simulink model "collision"  (R2018a)
settings: Solver=VariableStepAuto  StartTime=0.0  StopTime=120  FixedStep=0.01  MaxStep=.01  RelTol=1e-3
settings Model: Creator=U500304  LastModifiedBy=U500304
settings SolverCC: ZeroCrossAlgorithm=Adaptive
settings DataIOCC: SaveOutput=off  SaveTime=off
settings DebuggingCC: MaxConsecutiveZCsMsg=warning

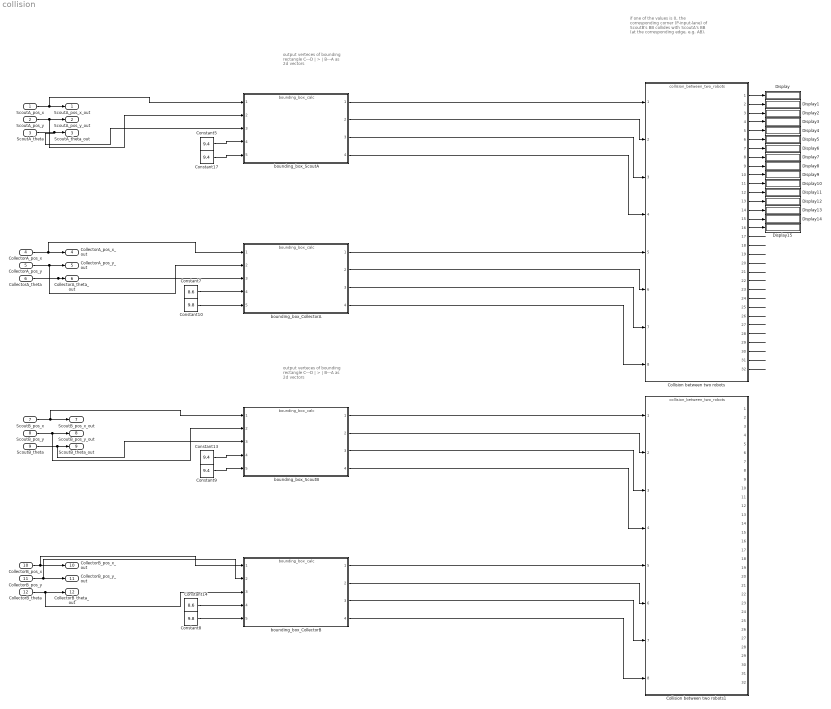
== system collision ==
  note: if one of the values is 0, the corresponding corner (P-input-lane) of ScoutB's BB collides with ScoutA's BB (at the corresponding edge, e.g. AB).
  note: output verteces of
      | bounding rectangle
      | C---D
      | |  >  |
      | B---A  as 2d vectors
  note: output verteces of
      | bounding rectangle
      | C---D
      | |  >  |
      | B---A  as 2d vectors
  ScoutA_pos_x : Inport  OutDataTypeStr=double  PortDimensions=1  SampleTime=0
  ScoutA_pos_y : Inport  Port=2  OutDataTypeStr=double  PortDimensions=1  SampleTime=0
  ScoutA_theta : Inport  Port=3  OutDataTypeStr=double  PortDimensions=1  SampleTime=0
  CollectorA_pos_x : Inport  Port=4  OutDataTypeStr=double  PortDimensions=1  SampleTime=0
  CollectorA_pos_y : Inport  Port=5  OutDataTypeStr=double  PortDimensions=1  SampleTime=0
  CollectorA_theta : Inport  Port=6  OutDataTypeStr=double  PortDimensions=1  SampleTime=0
  ScoutB_pos_x : Inport  Port=7  OutDataTypeStr=double  PortDimensions=1  SampleTime=0
  ScoutB_pos_y : Inport  Port=8  OutDataTypeStr=double  PortDimensions=1  SampleTime=0
  ScoutB_theta : Inport  Port=9  OutDataTypeStr=double  PortDimensions=1  SampleTime=0
  CollectorB_pos_x : Inport  Port=10  OutDataTypeStr=double  PortDimensions=1  SampleTime=0
  CollectorB_pos_y : Inport  Port=11  OutDataTypeStr=double  PortDimensions=1  SampleTime=0
  CollectorB_theta : Inport  Port=12  OutDataTypeStr=double  PortDimensions=1  SampleTime=0
  Collision between two robots : ModelReference  ModelNameDialog=collision_between_two_robots  SimulationMode=Normal  ModelReferenceVersion=1.665
  Collision between two robots1 : ModelReference  ModelNameDialog=collision_between_two_robots  SimulationMode=Normal  ModelReferenceVersion=1.665
  Constant10 : Constant  Value=9.8
  Constant{5,9,13,17} (4 alike) : Constant  Value=9.4
  Constant14 : Constant  Value=8.6
  Constant7 : Constant  Value=8.6
  Constant8 : Constant  Value=9.8
  Display{,1..15} (16 alike) : Display
  bounding_box_CollectorA : ModelReference  ModelNameDialog=bounding_box_calc  SimulationMode=Normal  ModelReferenceVersion=1.659
  bounding_box_CollectorB : ModelReference  ModelNameDialog=bounding_box_calc  SimulationMode=Normal  ModelReferenceVersion=1.659
  bounding_box_ScoutA : ModelReference  ModelNameDialog=bounding_box_calc  SimulationMode=Normal  ModelReferenceVersion=1.659
  bounding_box_ScoutB : ModelReference  ModelNameDialog=bounding_box_calc  SimulationMode=Normal  ModelReferenceVersion=1.659
  ScoutA_pos_x_out : Outport
  ScoutA_pos_y_out : Outport  Port=2
  ScoutA_theta_out : Outport  Port=3
  CollectorA_pos_x_out : Outport  Port=4
  CollectorA_pos_y_out : Outport  Port=5
  CollectorA_theta_out : Outport  Port=6
  ScoutB_pos_x_out : Outport  Port=7
  ScoutB_pos_y_out : Outport  Port=8
  ScoutB_theta_out : Outport  Port=9
  CollectorB_pos_x_out : Outport  Port=10
  CollectorB_pos_y_out : Outport  Port=11
  CollectorB_theta_out : Outport  Port=12
  wires:
  Constant10/1 -> bounding_box_CollectorA/5
  Constant17/1 -> bounding_box_ScoutA/5
  Constant7/1 -> bounding_box_CollectorA/4
  CollectorA_theta/1 -> bounding_box_CollectorA/3, CollectorA_theta_out/1
  Constant5/1 -> bounding_box_ScoutA/4
  CollectorA_pos_x/1 -> bounding_box_CollectorA/1, CollectorA_pos_x_out/1
  CollectorA_pos_y/1 -> bounding_box_CollectorA/2, CollectorA_pos_y_out/1
  bounding_box_ScoutA/1 -> Collision between two robots/1
  bounding_box_ScoutA/2 -> Collision between two robots/2
  bounding_box_ScoutA/3 -> Collision between two robots/3
  bounding_box_ScoutA/4 -> Collision between two robots/4
  bounding_box_CollectorA/1 -> Collision between two robots/5
  bounding_box_CollectorA/2 -> Collision between two robots/6
  bounding_box_CollectorA/3 -> Collision between two robots/7
  bounding_box_CollectorA/4 -> Collision between two robots/8
  bounding_box_CollectorB/4 -> Collision between two robots1/8
  bounding_box_CollectorB/3 -> Collision between two robots1/7
  bounding_box_CollectorB/2 -> Collision between two robots1/6
  bounding_box_CollectorB/1 -> Collision between two robots1/5
  bounding_box_ScoutB/4 -> Collision between two robots1/4
  bounding_box_ScoutB/3 -> Collision between two robots1/3
  bounding_box_ScoutB/2 -> Collision between two robots1/2
  bounding_box_ScoutB/1 -> Collision between two robots1/1
  Constant13/1 -> bounding_box_ScoutB/4
  Constant14/1 -> bounding_box_CollectorB/4
  Constant9/1 -> bounding_box_ScoutB/5
  Constant8/1 -> bounding_box_CollectorB/5
  ScoutA_pos_x/1 -> bounding_box_ScoutA/1, ScoutA_pos_x_out/1
  ScoutA_pos_y/1 -> bounding_box_ScoutA/2, ScoutA_pos_y_out/1
  ScoutA_theta/1 -> bounding_box_ScoutA/3, ScoutA_theta_out/1
  ScoutB_theta/1 -> bounding_box_ScoutB/3, ScoutB_theta_out/1
  ScoutB_pos_y/1 -> bounding_box_ScoutB/2, ScoutB_pos_y_out/1
  ScoutB_pos_x/1 -> bounding_box_ScoutB/1, ScoutB_pos_x_out/1
  CollectorB_theta/1 -> bounding_box_CollectorB/3, CollectorB_theta_out/1
  CollectorB_pos_y/1 -> bounding_box_CollectorB/2, CollectorB_pos_y_out/1
  CollectorB_pos_x/1 -> bounding_box_CollectorB/1, CollectorB_pos_x_out/1
  Collision between two robots/1 -> Display/1
  Collision between two robots/2 -> Display1/1
  Collision between two robots/3 -> Display2/1
  Collision between two robots/4 -> Display3/1
  Collision between two robots/6 -> Display5/1
  Collision between two robots/5 -> Display4/1
  Collision between two robots/7 -> Display6/1
  Collision between two robots/8 -> Display7/1
  Collision between two robots/9 -> Display8/1
  Collision between two robots/10 -> Display9/1
  Collision between two robots/11 -> Display10/1
  Collision between two robots/12 -> Display11/1
  Collision between two robots/13 -> Display12/1
  Collision between two robots/14 -> Display13/1
  Collision between two robots/15 -> Display14/1
  Collision between two robots/16 -> Display15/1
  Collision between two robots/17 -> ?
  Collision between two robots/18 -> ?
  Collision between two robots/19 -> ?
  Collision between two robots/20 -> ?
  Collision between two robots/21 -> ?
  Collision between two robots/22 -> ?
  Collision between two robots/23 -> ?
  Collision between two robots/24 -> ?
  Collision between two robots/25 -> ?
  Collision between two robots/26 -> ?
  Collision between two robots/27 -> ?
  Collision between two robots/28 -> ?
  Collision between two robots/29 -> ?
  Collision between two robots/30 -> ?
  Collision between two robots/31 -> ?
  Collision between two robots/32 -> ?
